simulink library "project3Library"  (R2020a)
settings: Solver=VariableStepAuto  StartTime=0.0  StopTime=10.0  RelTol=1e-3
settings Model: Creator=ggparker  LastModifiedBy=ggparker
settings SFSimCC: CustomCodeUndefinedFunction=UseInterfaceOnly

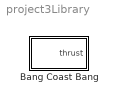
== system project3Library ==
  Bang Coast Bang : Subsystem  mask{amp=0, tStart=1, tPW=2, tCoast=0}
      mask prompts: amp "Thrust Amp (N)"; tStart "Start Time (sec)"; tPW "Pulse Width (sec)"; tCoast "Coast Time (sec)"
      settings: AttributesFormatString=t = %<tStart>, A = %<amp>

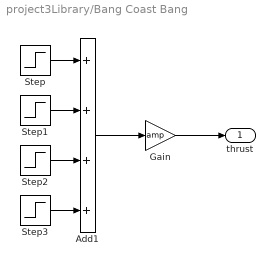
== system project3Library/Bang Coast Bang ==
  Add1 : Sum  Inputs=++++
  Gain : Gain  Gain=amp
  Step : Step  Time=tStart  SampleTime=0
  Step1 : Step  Time=tStart+tPW  After=-1  SampleTime=0
  Step2 : Step  Time=tStart+tPW+tCoast  After=-1  SampleTime=0
  Step3 : Step  Time=tStart+2*tPW+tCoast  SampleTime=0
  thrust : Outport  VectorParamsAs1DForOutWhenUnconnected=off
  wires:
  Step/1 -> Add1/1
  Step1/1 -> Add1/2
  Step2/1 -> Add1/3
  Step3/1 -> Add1/4
  Add1/1 -> Gain/1
  Gain/1 -> thrust/1
